simulink model "Problem1"  (R2020b)
settings: Solver=VariableStepAuto  StartTime=0.0  StopTime=10.0  RelTol=1e-3
model workspace (MAT data in the model file):
  M1 = Simulink.Parameter
  M1.Value = 1000
  M1.DataType = 'auto'
  M1.Dimensions = [1 1]
  b = Simulink.Parameter
  b.Value = 50
  b.DataType = 'auto'
  b.Dimensions = [1 1]
  k1 = Simulink.Parameter
  k1.Value = 50
  k1.DataType = 'auto'
  k1.Dimensions = [1 1]
settings Model: OrderedModelArguments=off  Creator=ASUS  LastModifiedBy=ASUS

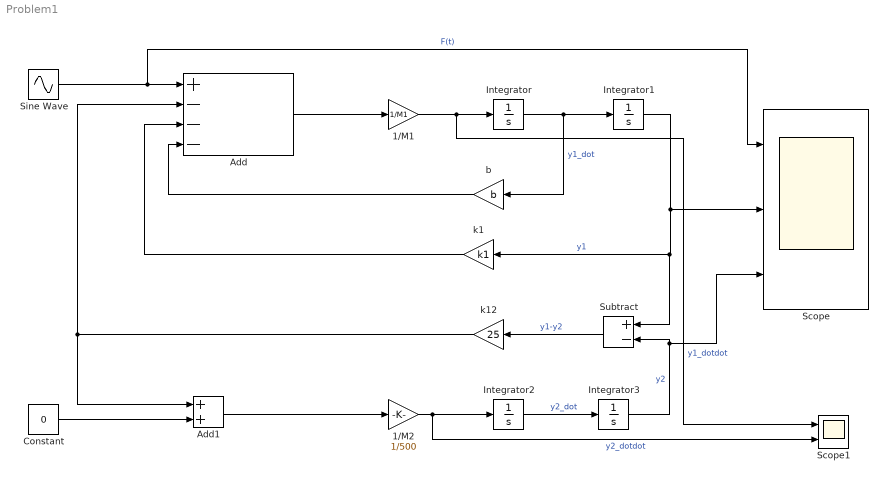
== system Problem1 ==
  1/M1 : Gain  Gain=1/M1
  1/M2 : Gain  Gain=1/500
  Add : Sum  Inputs=+---
  Add1 : Sum
  Constant : Constant  Value=0
  Integrator{,1..3} (4 alike) : Integrator
  Scope : Scope  NumInputPorts=3
  Scope1 : Scope  NumInputPorts=2
  Sine Wave : Sin  Amplitude=2  Frequency=10  SampleTime=.01
  Subtract : Sum  Inputs=+-
  b : Gain  Gain=b
  k1 : Gain  Gain=k1
  k12 : Gain  Gain=25
  wires:
  Sine Wave/1 -> Scope/1, Add/1  "F(t)"
  Add/1 -> 1/M1/1
  Integrator/1 -> Integrator1/1, b/1  "y1_dot"
  b/1 -> Add/4
  Integrator1/1 -> Subtract/1, k1/1, Scope/2  "y1"
  k1/1 -> Add/3
  Integrator2/1 -> Integrator3/1  "y2_dot"
  Constant/1 -> Add1/2
  Integrator3/1 -> Scope/3, Subtract/2  "y2"
  k12/1 -> Add/2, Add1/1
  Subtract/1 -> k12/1  "y1-y2"
  Add1/1 -> 1/M2/1
  1/M2/1 -> Scope1/2, Integrator2/1  "y2_dotdot"
  1/M1/1 -> Scope1/1, Integrator/1  "y1_dotdot"
